simulink model "MPC_VSC_AS"  (R2022b)
settings: Solver=ode4  StartTime=0.0  StopTime=20  FixedStep=1e-3  RelTol=1e-3  EnableMultiTasking=on
values from neighbouring files (symbols this model uses):
  Dt = 0.01    [MAIN_AS.m]
  g = 9.81    [MAIN_AS.m]
  i_steer = 15.4    [MAIN_AS.m]
  Kus = m_f/Caf-m_r/Car    (= 0.00219239766082)    [MAIN_AS.m]
  L = 2.79    [MAIN_AS.m]
  mu = 1    [MAIN_AS.m]
  N = 20    [MAIN_AS.m]
  noise = 0    [MAIN_AS.m]
  tau = 0.09    [MAIN_AS.m]
  V_ref = 60/3.6    (= 16.6666666667)    [MAIN_AS.m]
  wn = 11    [MAIN_AS.m]
  xi = 0.7    [MAIN_AS.m]
undefined symbols (not defined in the file or in its folder): MPC_constraints, MPC_weights, par
libraries: simulink x2
settings Model: Creator=bshyrokau  LastModifiedBy=xippa
settings SolverCC: AlgebraicLoopSolver=TrustRegion
settings DataIOCC: SaveOutput=off  SignalLogging=off  DSMLogging=off  SaveTime=off  ReturnWorkspaceOutputs=off
settings OptimizationCC: LifeSpan=inf
settings DebuggingCC: UnconnectedInputMsg=warning  UnconnectedOutputMsg=warning  UnconnectedLineMsg=warning  AllowSymbolicDim=off  SFUnexpectedBacktrackingDiag=warning  SFNoUnconditionalDefaultTransitionDiag=warning  SFExecutionAtInitializationDiag=none  ArithmeticOperatorsInVariantConditions=warning
settings ModelReferenceCC: EnableRefExpFcnMdlSchedulingChecks=on  PropagateSignalLabelsOutOfModel=off
settings SFSimCC: SimUseLocalCustomCode=off  CustomCodeUndefinedFunction=UseInterfaceOnly
settings RTWCC: RTWUseLocalCustomCode=off  DLArmComputeVersion=19.05
settings CodeAppCC: StateflowObjectComments=on
settings GRTTargetCC: TargetLangStandard=C89/C90 (ANSI)
settings ConfigComp: CovMetricSettings=dw  CovSaveCumulativeToWorkspaceVar=on  CovSaveSingleToWorkspaceVar=on  CovExternalEMLEnable=off
settings SimscapeCC: SimscapeNormalizeSystem=off
settings ConfigurationSet: Description=SimMechanics 2G

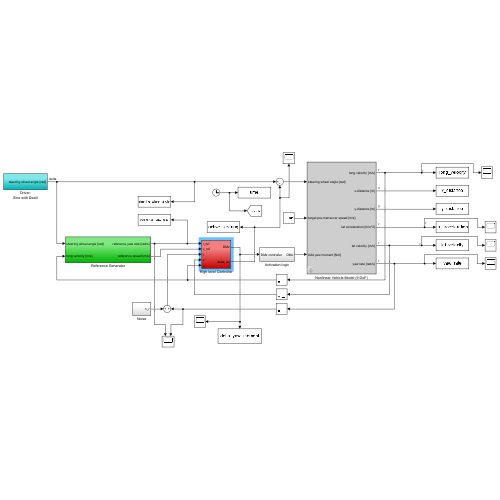
[thumbnail: Simulink's stored preview of the top-level diagram]
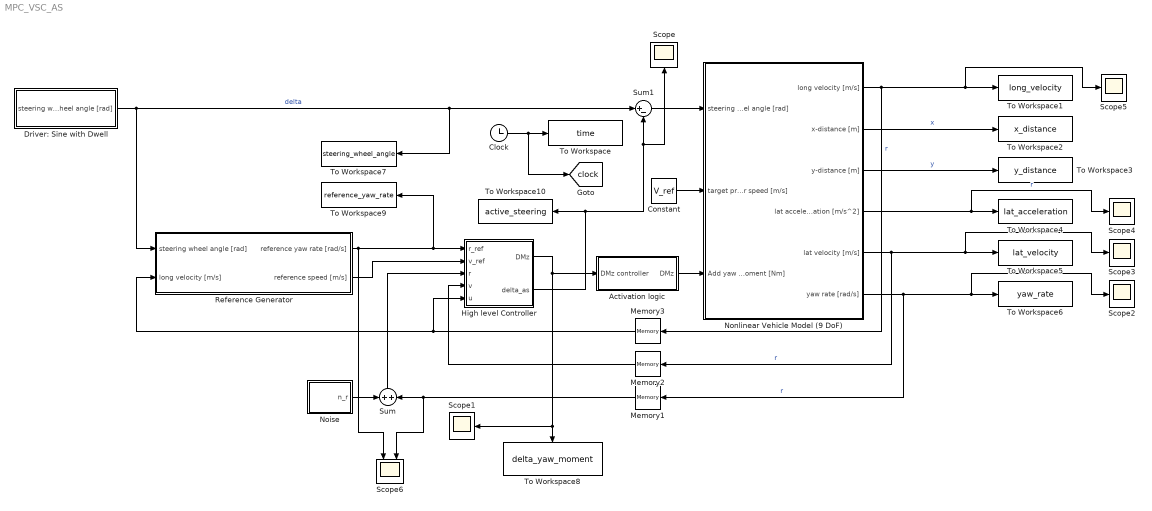
== system MPC_VSC_AS ==
  Activation logic : Subsystem
  Clock : Clock
  Constant : Constant  Value=V_ref
  Driver: Sine with Dwell : Subsystem
  High level Controller : Subsystem
  Memory1 : Memory
  Memory2 : Memory
  Memory3 : Memory
  Noise : Subsystem
  Nonlinear Vehicle Model (9 DoF) : Subsystem
      mask help: Simulink:masks:GenSFuncDesc_MD
      mask Help: eval('feval(''rtwprivate'',''rtwhelpview'',''rtw_sfcn_block'')');
  Reference Generator : Subsystem
  Scope{,1..5} (6 alike) : Scope
  Scope6 : Scope  NumInputPorts=2
  Sum : Sum  Inputs=+|+
  Sum1 : Sum  Inputs=|+-
  To Workspace : ToWorkspace  VariableName=time  SampleTime=-1
  To Workspace1 : ToWorkspace  VariableName=long_velocity  SampleTime=-1
  To Workspace10 : ToWorkspace  VariableName=active_steering  SampleTime=-1
  To Workspace2 : ToWorkspace  VariableName=x_distance  SampleTime=-1
  To Workspace3 : ToWorkspace  VariableName=y_distance  SampleTime=-1
  To Workspace4 : ToWorkspace  VariableName=lat_acceleration  SampleTime=-1
  To Workspace5 : ToWorkspace  VariableName=lat_velocity  SampleTime=-1
  To Workspace6 : ToWorkspace  VariableName=yaw_rate  SampleTime=-1
  To Workspace7 : ToWorkspace  VariableName=steering_wheel_angle  SampleTime=-1
  To Workspace8 : ToWorkspace  VariableName=delta_yaw_moment  SampleTime=-1
  To Workspace9 : ToWorkspace  VariableName=reference_yaw_rate  SampleTime=-1
  tag scope: clock=global
  wires:
  Driver: Sine with Dwell/1(steering wheel angle [rad]) -> Sum1/1, To Workspace7/1, Reference Generator/1(steering wheel angle [rad])  "delta"
  Reference Generator/1(reference yaw rate [rad/s]) -> High level Controller/1(r_ref), To Workspace9/1, Scope6/1
  Nonlinear Vehicle Model (9 DoF)/6(yaw rate [rad/s]) -> Scope2/1, To Workspace6/1, Memory1/1  "r"
  Nonlinear Vehicle Model (9 DoF)/2(x-distance [m]) -> To Workspace2/1  "x"
  Nonlinear Vehicle Model (9 DoF)/3(y-distance [m]) -> To Workspace3/1  "y"
  Constant/1 -> Nonlinear Vehicle Model (9 DoF)/2(target pre-maneuver speed [m/s])
  Clock/1 -> To Workspace/1, [clock]
  Memory1/1 -> Scope6/2, Sum/2
  Sum/1 -> High level Controller/3(r)
  Activation logic/1(DMz) -> Nonlinear Vehicle Model (9 DoF)/3(Add yaw moment [Nm])
  Noise/1(n_r) -> Sum/1
  Memory2/1 -> High level Controller/4(v)
  Memory3/1 -> High level Controller/5(u), Reference Generator/2(long velocity [m/s])
  Reference Generator/2(reference speed [m/s]) -> High level Controller/2(v_ref)
  High level Controller/1(DMz) -> Activation logic/1(DMz controller), Scope1/1, To Workspace8/1
  High level Controller/2(delta_as) -> To Workspace10/1, Scope/1, Sum1/2
  Sum1/1 -> Nonlinear Vehicle Model (9 DoF)/1(steering wheel angle [rad])
  Nonlinear Vehicle Model (9 DoF)/5(lat velocity [m/s]) -> Scope3/1, To Workspace5/1, Memory2/1  "r"
  Nonlinear Vehicle Model (9 DoF)/4(lat acceleration [m/s^2]) -> Scope4/1, To Workspace4/1  "r"
  Nonlinear Vehicle Model (9 DoF)/1(long velocity [m/s]) -> Scope5/1, To Workspace1/1, Memory3/1  "r"

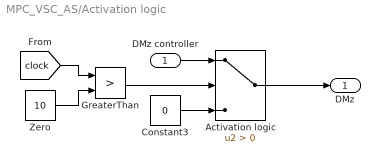
== system MPC_VSC_AS/Activation logic ==
  DMz controller : Inport
  Activation logic : Switch  Criteria=u2 > Threshold  SaturateOnIntegerOverflow=off  InputSameDT=off
  Constant3 : Constant  Value=0
  GreaterThan : RelationalOperator  Operator=>  OutDataTypeStr=boolean  RndMeth=Simplest  InputSameDT=off
  Zero : Constant  Value=10  OutDataTypeStr=Inherit: Inherit via back propagation
  DMz : Outport
  wires:
  [clock] -> GreaterThan/1
  GreaterThan/1 -> Activation logic/2
  Activation logic/1 -> DMz/1
  DMz controller/1 -> Activation logic/1
  Zero/1 -> GreaterThan/2
  Constant3/1 -> Activation logic/3

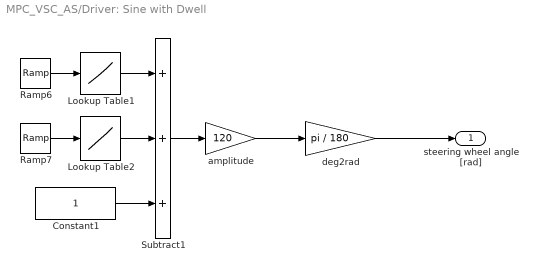
== system MPC_VSC_AS/Driver: Sine with Dwell ==
  Constant1 : Constant
  Lookup Table1 : Lookup  InputValues=[0:0.1:3*pi/2 3*pi/2+eps]*0.7  Table=sin([0:0.1:3*pi/2 3*pi/2+eps])  LookUpMeth=Interpolation-Use End Values  SaturateOnIntegerOverflow=off
  Lookup Table2 : Lookup  InputValues=[3*pi/2:0.1:2*pi 2*pi+eps]*0.7  Table=sin([3*pi/2:0.1:2*pi 2*pi+eps])  LookUpMeth=Interpolation-Use End Values  SaturateOnIntegerOverflow=off
  Ramp6 : simulink/Sources/Ramp  slope=pi  start=10  InitialOutput=0
  Ramp7 : simulink/Sources/Ramp  slope=pi  start=10+0.5  InitialOutput=0
  Subtract1 : Sum  Inputs=+++
  amplitude : Gain  Gain=120
  deg2rad : Gain  Gain=pi / 180
  steering wheel angle [rad] : Outport  VectorParamsAs1DForOutWhenUnconnected=off
  wires:
  Ramp6/1 -> Lookup Table1/1
  Ramp7/1 -> Lookup Table2/1
  Lookup Table2/1 -> Subtract1/2
  Lookup Table1/1 -> Subtract1/1
  Constant1/1 -> Subtract1/3
  Subtract1/1 -> amplitude/1
  amplitude/1 -> deg2rad/1
  deg2rad/1 -> steering wheel angle [rad]/1

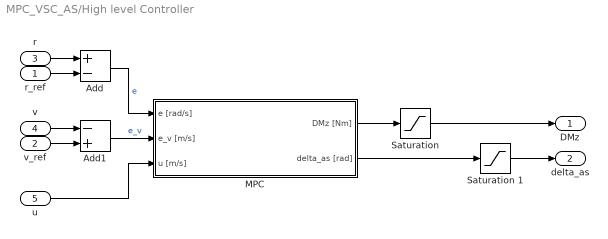
== system MPC_VSC_AS/High level Controller ==
  r_ref : Inport
  v_ref : Inport  Port=2
  r : Inport  Port=3
  v : Inport  Port=4
  u : Inport  Port=5
  Add : Sum  Inputs=+-
  Add1 : Sum  Inputs=-+
  MPC : Subsystem
  "Saturation " : Saturate  UpperLimit=10000  LowerLimit=-10000
  Saturation 1 : Saturate  UpperLimit=deg2rad(10)  LowerLimit=-deg2rad(10)
  DMz : Outport  VectorParamsAs1DForOutWhenUnconnected=off
  delta_as : Outport  Port=2  VectorParamsAs1DForOutWhenUnconnected=off
  wires:
  r_ref/1 -> Add/2
  "Saturation "/1 -> DMz/1
  Add/1 -> MPC/1(e [rad/s])  "e"
  r/1 -> Add/1
  v/1 -> Add1/1
  u/1 -> MPC/3(u [m/s])
  MPC/1(DMz [Nm]) -> "Saturation "/1
  v_ref/1 -> Add1/2
  Add1/1 -> MPC/2(e_v [m/s])  "e_v"
  MPC/2(delta_as [rad]) -> Saturation 1/1
  Saturation 1/1 -> delta_as/1

== system MPC_VSC_AS/Noise ==
  Constant1 : Constant  Value=0
  Constant2 : Constant  Value=noise
  Switch : Switch  Criteria=u2 > Threshold  SaturateOnIntegerOverflow=off  InputSameDT=off
  Uniform Random Number : UniformRandomNumber  Minimum=-deg2rad(0.5)  Maximum=deg2rad(0.5)  SampleTime=0.001
  n_r : Outport
  wires:
  Switch/1 -> n_r/1
  Constant2/1 -> Switch/2
  Constant1/1 -> Switch/3
  Uniform Random Number/1 -> Switch/1

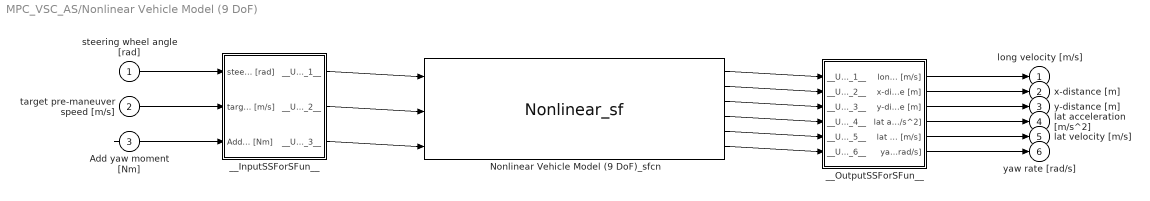
== system MPC_VSC_AS/Nonlinear Vehicle Model (9 DoF) ==
  steering wheel angle [rad] : Inport
  target pre-maneuver speed [m/s] : Inport  Port=2
  Add yaw moment [Nm] : Inport  Port=3
  Nonlinear Vehicle Model (9 DoF)_sfcn : S-Function  FunctionName=Nonlinear_sf  SFunctionModules=""  SFunctionDeploymentMode=off  EnableBusSupport=off  mask{rtw_sf_name=Nonlinear_sf, showVar=off}
      mask prompts: rtw_sf_name "Simulink:masks:GenSFuncName_MP"; showVar "Simulink:masks:GenSFuncShowModuleList_MP"
      mask help: Simulink:masks:GenSFuncDesc_MD
      mask init:
      | displist = '';
      | if ~strcmp(get_param(gcb, 'FunctionName'), rtw_sf_name);
      |   set_param(gcb, 'FunctionName', rtw_sf_name);
      | end
      | % Check if we are generating code
      | rtw_mode = false;
      | if strcmpi(get_param(bdroot(gcb),'SimulationStatus'),'Initializing')
      | 	rtw_mode = strcmpi(get_param(bdroot(gcb),'BuildingRTWCode'),'on') && ...
      | 		~strcmpi(get_param(bdroot(gcb),'TargetStyle'),'SimulationTarget');
      | end
      | if showVar || rtw_mode
      | 	if exist('rtwsfunc') == 2 | exist('rtwsfunc') == 6
      | 		tmplist = rtwsfunc(rtw_sf_name,gcb);
      | 		tmplist = DAStudio.message('Simulink:masks:GenSFuncListOfModules_IC', tmplist);
      | 	elseif showVar
      | 		tmplist1 = DAStudio.message('Simulink:masks:GenSFuncListOfModules_IC', '');
      |         tmplist2 = DAStudio.message('Simulink:masks:GenSFuncNotLicensed_IC');
      |         tmplist = [tmplist1 tmplist2];
      |  	end
      | end
      | if showVar
      |   displist = tmplist;
      | end
      settings: CopyFcn=|
      | if ~strcmp(get_param(gcb,'Linkstatus'),'none') && ...
      | ~strcmp(get_param(gcb,'Linkstatus'),'implicit')
      |   set_param(gcb,'LinkStatus','none');
      | end
      mask Help: eval('feval(''rtwprivate'',''rtwhelpview'',''rtw_sfcn_block'')');
      mask Display:
      | port_label('input',1,'steering wheel angle [rad]');
      | port_label('input',2,'target pre-maneuver speed [m/s]');
      | port_label('input',3,'Add yaw moment [Nm]');
      | port_label('output',1,'long velocity [m/s]');
      | port_label('output',2,'x-distance [m]');
      | port_label('output',3,'y-distance [m]');
      | port_label('output',4,'lat acceleration [m/s^2]');
      | port_label('output',5,'lat velocity [m/s]');
      | port_label('output',6,'yaw rate [rad/s]');
  __InputSSForSFun__ : Subsystem
  __OutputSSForSFun__ : Subsystem
  long velocity [m/s] : Outport  VectorParamsAs1DForOutWhenUnconnected=off
  x-distance [m] : Outport  Port=2  VectorParamsAs1DForOutWhenUnconnected=off
  y-distance [m] : Outport  Port=3  VectorParamsAs1DForOutWhenUnconnected=off
  lat acceleration [m/s^2] : Outport  Port=4  VectorParamsAs1DForOutWhenUnconnected=off
  lat velocity [m/s] : Outport  Port=5  VectorParamsAs1DForOutWhenUnconnected=off
  yaw rate [rad/s] : Outport  Port=6  VectorParamsAs1DForOutWhenUnconnected=off
  wires:
  steering wheel angle [rad]/1 -> __InputSSForSFun__/1(steering wheel angle [rad])
  target pre-maneuver speed [m/s]/1 -> __InputSSForSFun__/2(target pre-maneuver speed [m/s])
  Add yaw moment [Nm]/1 -> __InputSSForSFun__/3(Add yaw moment [Nm])
  __InputSSForSFun__/1(__UniqueOutportName__1__) -> Nonlinear Vehicle Model (9 DoF)_sfcn/1
  __InputSSForSFun__/2(__UniqueOutportName__2__) -> Nonlinear Vehicle Model (9 DoF)_sfcn/2
  __InputSSForSFun__/3(__UniqueOutportName__3__) -> Nonlinear Vehicle Model (9 DoF)_sfcn/3
  Nonlinear Vehicle Model (9 DoF)_sfcn/1 -> __OutputSSForSFun__/1(__UniqueInportName__1__)
  Nonlinear Vehicle Model (9 DoF)_sfcn/2 -> __OutputSSForSFun__/2(__UniqueInportName__2__)
  Nonlinear Vehicle Model (9 DoF)_sfcn/3 -> __OutputSSForSFun__/3(__UniqueInportName__3__)
  Nonlinear Vehicle Model (9 DoF)_sfcn/4 -> __OutputSSForSFun__/4(__UniqueInportName__4__)
  Nonlinear Vehicle Model (9 DoF)_sfcn/5 -> __OutputSSForSFun__/5(__UniqueInportName__5__)
  Nonlinear Vehicle Model (9 DoF)_sfcn/6 -> __OutputSSForSFun__/6(__UniqueInportName__6__)
  __OutputSSForSFun__/1(long velocity [m/s]) -> long velocity [m/s]/1
  __OutputSSForSFun__/2(x-distance [m]) -> x-distance [m]/1
  __OutputSSForSFun__/3(y-distance [m]) -> y-distance [m]/1
  __OutputSSForSFun__/4(lat acceleration [m/s^2]) -> lat acceleration [m/s^2]/1
  __OutputSSForSFun__/5(lat velocity [m/s]) -> lat velocity [m/s]/1
  __OutputSSForSFun__/6(yaw rate [rad/s]) -> yaw rate [rad/s]/1

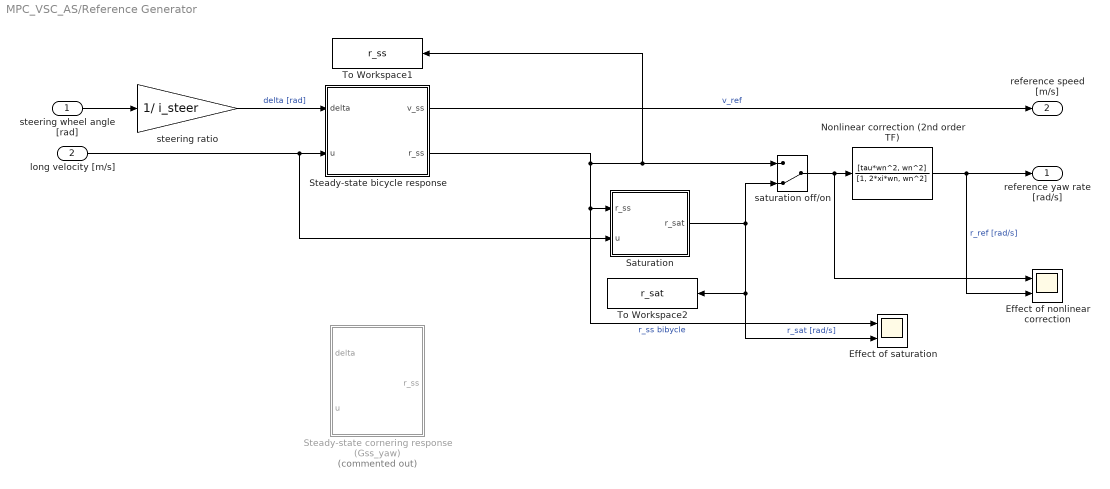
== system MPC_VSC_AS/Reference Generator ==
  steering wheel angle [rad] : Inport
  long velocity [m/s] : Inport  Port=2
  Effect of nonlinear correction : Scope  NumInputPorts=2
  Effect of saturation : Scope  NumInputPorts=2
  Nonlinear correction (2nd order TF) : TransferFcn  Numerator=[tau*wn^2, wn^2]  Denominator=[1, 2*xi*wn, wn^2]
  Saturation : Subsystem
  Steady-state bicycle response : MATLAB Function  TreatAsAtomicUnit=on
  Steady-state cornering response (Gss_yaw) : Subsystem  Commented=on
  To Workspace1 : ToWorkspace  VariableName=r_ss  SampleTime=-1
  To Workspace2 : ToWorkspace  VariableName=r_sat  SampleTime=-1
  saturation off/on : ManualSwitch  CurrentSetting=0
  steering ratio : Gain  Gain=1/ i_steer
  reference yaw rate [rad/s] : Outport  VectorParamsAs1DForOutWhenUnconnected=off
  reference speed [m/s] : Outport  Port=2  VectorParamsAs1DForOutWhenUnconnected=off
  wires:
  steering wheel angle [rad]/1 -> steering ratio/1
  steering ratio/1 -> Steady-state bicycle response/1(delta)  "delta [rad]"
  Steady-state bicycle response/2(r_ss) -> To Workspace1/1, saturation off/on/1, Effect of saturation/1, Saturation/1(r_ss)  "r_ss bibycle"
  Nonlinear correction (2nd order TF)/1 -> Effect of nonlinear correction/2, reference yaw rate [rad/s]/1  "r_ref [rad/s]"
  Saturation/1(r_sat) -> Effect of saturation/2, To Workspace2/1, saturation off/on/2  "r_sat [rad/s]"
  long velocity [m/s]/1 -> Saturation/2(u), Steady-state bicycle response/2(u)
  Steady-state bicycle response/1(v_ss) -> reference speed [m/s]/1  "v_ref"
  saturation off/on/1 -> Effect of nonlinear correction/1, Nonlinear correction (2nd order TF)/1

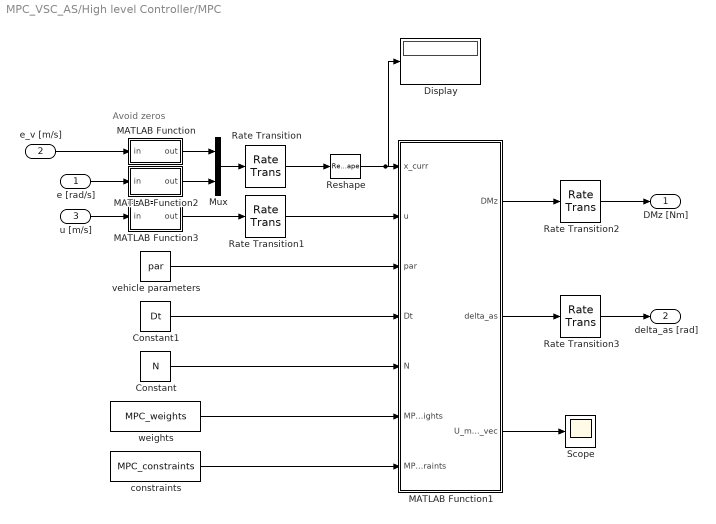
== system MPC_VSC_AS/High level Controller/MPC ==
  note: Avoid zeros
  e [rad/s] : Inport
  e_v [m/s] : Inport  Port=2
  u [m/s] : Inport  Port=3
  Constant : Constant  Value=N
  Constant1 : Constant  Value=Dt
  Display : Display
  MATLAB Function : MATLAB Function  TreatAsAtomicUnit=on
  MATLAB Function1 : MATLAB Function  TreatAsAtomicUnit=on
  MATLAB Function2 : MATLAB Function  TreatAsAtomicUnit=on
  MATLAB Function3 : MATLAB Function  TreatAsAtomicUnit=on
  Mux : Mux  Inputs=2
  Rate Transition : RateTransition  OutPortSampleTime=Dt
  Rate Transition1 : RateTransition  OutPortSampleTime=Dt
  Rate Transition2 : RateTransition  OutPortSampleTime=1e-3
  Rate Transition3 : RateTransition  OutPortSampleTime=1e-3
  Reshape : Reshape  OutputDimensionality=Customize  OutputDimensions=[2,1]
  Scope : Scope
  constraints : Constant  Value=MPC_constraints  OutDataTypeStr=Bus: constraintsBus
  vehicle parameters : Constant  Value=par  OutDataTypeStr=Bus: parBus
  weights : Constant  Value=MPC_weights  OutDataTypeStr=Bus: weightsBus
  DMz [Nm] : Outport
  delta_as [rad] : Outport  Port=2
  wires:
  e [rad/s]/1 -> MATLAB Function2/1(in)
  MATLAB Function1/1(DMz) -> Rate Transition2/1
  e_v [m/s]/1 -> MATLAB Function/1(in)
  Mux/1 -> Rate Transition/1
  vehicle parameters/1 -> MATLAB Function1/3(par)
  Constant/1 -> MATLAB Function1/5(N)
  Constant1/1 -> MATLAB Function1/4(Dt)
  u [m/s]/1 -> MATLAB Function3/1(in)
  weights/1 -> MATLAB Function1/6(MPC_weights)
  constraints/1 -> MATLAB Function1/7(MPC_constraints)
  Rate Transition1/1 -> MATLAB Function1/2(u)
  Rate Transition2/1 -> DMz [Nm]/1
  MATLAB Function/1(out) -> Mux/1
  MATLAB Function2/1(out) -> Mux/2
  MATLAB Function3/1(out) -> Rate Transition1/1
  Rate Transition3/1 -> delta_as [rad]/1
  MATLAB Function1/2(delta_as) -> Rate Transition3/1
  Rate Transition/1 -> Reshape/1
  Reshape/1 -> Display/1, MATLAB Function1/1(x_curr)
  MATLAB Function1/3(U_min_vec) -> Scope/1

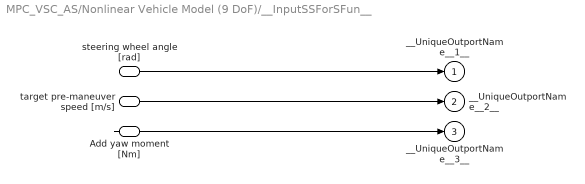
== system MPC_VSC_AS/Nonlinear Vehicle Model (9 DoF)/__InputSSForSFun__ ==
  steering wheel angle [rad] : Inport
  target pre-maneuver speed [m/s] : Inport  Port=2
  Add yaw moment [Nm] : Inport  Port=3
  __UniqueOutportName__1__ : Outport
  __UniqueOutportName__2__ : Outport  Port=2
  __UniqueOutportName__3__ : Outport  Port=3
  wires:
  steering wheel angle [rad]/1 -> __UniqueOutportName__1__/1
  target pre-maneuver speed [m/s]/1 -> __UniqueOutportName__2__/1
  Add yaw moment [Nm]/1 -> __UniqueOutportName__3__/1

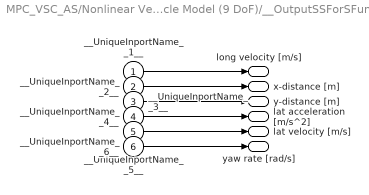
== system MPC_VSC_AS/Nonlinear Vehicle Model (9 DoF)/__OutputSSForSFun__ ==
  __UniqueInportName__1__ : Inport
  __UniqueInportName__2__ : Inport  Port=2
  __UniqueInportName__3__ : Inport  Port=3
  __UniqueInportName__4__ : Inport  Port=4
  __UniqueInportName__5__ : Inport  Port=5
  __UniqueInportName__6__ : Inport  Port=6
  long velocity [m/s] : Outport  VectorParamsAs1DForOutWhenUnconnected=off
  x-distance [m] : Outport  Port=2  VectorParamsAs1DForOutWhenUnconnected=off
  y-distance [m] : Outport  Port=3  VectorParamsAs1DForOutWhenUnconnected=off
  lat acceleration [m/s^2] : Outport  Port=4  VectorParamsAs1DForOutWhenUnconnected=off
  lat velocity [m/s] : Outport  Port=5  VectorParamsAs1DForOutWhenUnconnected=off
  yaw rate [rad/s] : Outport  Port=6  VectorParamsAs1DForOutWhenUnconnected=off
  wires:
  __UniqueInportName__1__/1 -> long velocity [m/s]/1
  __UniqueInportName__2__/1 -> x-distance [m]/1
  __UniqueInportName__3__/1 -> y-distance [m]/1
  __UniqueInportName__4__/1 -> lat acceleration [m/s^2]/1
  __UniqueInportName__5__/1 -> lat velocity [m/s]/1
  __UniqueInportName__6__/1 -> yaw rate [rad/s]/1

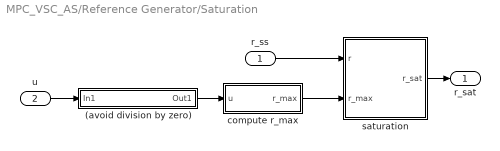
== system MPC_VSC_AS/Reference Generator/Saturation ==
  r_ss : Inport
  u : Inport  Port=2
  (avoid division by zero) : Subsystem
  compute r_max : Subsystem
  saturation : MATLAB Function  TreatAsAtomicUnit=on
  r_sat : Outport
  wires:
  compute r_max/1(r_max) -> saturation/2(r_max)
  saturation/1(r_sat) -> r_sat/1
  r_ss/1 -> saturation/1(r)
  u/1 -> (avoid division by zero)/1(In1)
  (avoid division by zero)/1(Out1) -> compute r_max/1(u)

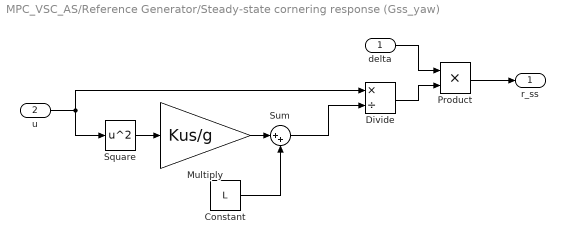
== system MPC_VSC_AS/Reference Generator/Steady-state cornering response (Gss_yaw) ==
  delta : Inport
  u : Inport  Port=2
  Constant : Constant  Value=L
  Divide : Product  Inputs=*/
  Multiply : Gain  Gain=Kus/g
  Product : Product
  Square : Math  Operator=square
  Sum : Sum  Inputs=|++
  r_ss : Outport
  wires:
  u/1 -> Square/1, Divide/1
  Square/1 -> Multiply/1
  Multiply/1 -> Sum/1
  Constant/1 -> Sum/2
  Sum/1 -> Divide/2
  delta/1 -> Product/1
  Divide/1 -> Product/2
  Product/1 -> r_ss/1

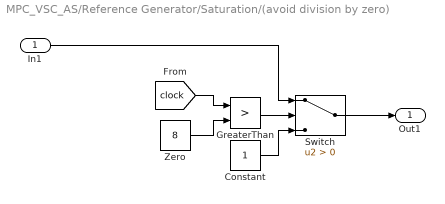
== system MPC_VSC_AS/Reference Generator/Saturation/(avoid division by zero) ==
  In1 : Inport
  Constant : Constant
  GreaterThan : RelationalOperator  Operator=>  OutDataTypeStr=boolean  RndMeth=Simplest  InputSameDT=off
  Switch : Switch  Criteria=u2 > Threshold  SaturateOnIntegerOverflow=off  InputSameDT=off
  Zero : Constant  Value=8  OutDataTypeStr=Inherit: Inherit via back propagation
  Out1 : Outport
  wires:
  Constant/1 -> Switch/3
  [clock] -> GreaterThan/1
  GreaterThan/1 -> Switch/2
  Switch/1 -> Out1/1
  In1/1 -> Switch/1
  Zero/1 -> GreaterThan/2

== system MPC_VSC_AS/Reference Generator/Saturation/compute r_max ==
  u : Inport
  Constant : Constant  Value=0.85*mu*g
  Divide : Product  Inputs=*/
  r_max : Outport
  wires:
  Constant/1 -> Divide/1
  Divide/1 -> r_max/1
  u/1 -> Divide/2

== matlab function MPC_VSC_AS/Reference Generator/Steady-state bicycle response ==
  data: v_ss output; delta input; u input; r_ss output
function [v_ss,r_ss]=ssBicycle(delta,u)

% Parameters
m = 1380;       % vehicle mass [Kg]    
L = 2.79;       % wheelbase [m]
lf = 1.384;     % distance from front axle to CoG [m]
lr = L-lf;      % distance from rear axle to CoG [m]
Caf = 120000;   % front axle cornering stiffness
Car = 190000;   % rear axle cornering stiffness
Iz = 2634.5;    % body inertia around z-axis [Kg m^2]

% Compute A matrix
A=zeros(2,2);
A(1,1)=-(Caf+Car)/(m*u);
A(1,2)=(lr*Car-lf*Caf)/(m*u)-u;
A(2,1)=(lr*Car-lf*Caf)/(Iz*u);
A(2,2)=-(lf^2*Caf+lr^2*Car)/(Iz*u);

% Compute B vector
B=[Caf/m Caf*lf/Iz]';

% Solve steady-state bicycle
x_ref=-A\(B*delta);
v_ss=x_ref(1);
r_ss=x_ref(2);

if any(isnan(x_ref))
    v_ss=0;
    r_ss=0;
end

end

== matlab function MPC_VSC_AS/Reference Generator/Saturation/saturation ==
  data: r input; r_sat output; r_max input
function r_sat=sat(r,r_max)

if r>r_max
    r_sat=r_max;
elseif r<-r_max
    r_sat=-r_max;
else
    r_sat=r;
end

end

== matlab function MPC_VSC_AS/High level Controller/MPC/MATLAB Function ==
  data: in input; out output
function out=fcn(in)

if in==0
    out=0.001;
else
    out=in;
end

end

== matlab function MPC_VSC_AS/High level Controller/MPC/MATLAB Function1 ==
  data: x_curr input; u input; par input; Dt input; DMz output; N input; MPC_weights input; MPC_constraints input; delta_as output; U_min_vec output
function [DMz, delta_as, U_min_vec] = MPC(x_curr,u,par,Dt,N,MPC_weights,MPC_constraints)
% Extract relevant parameters from structs
Iz=par.Iz;
Caf=par.Caf;
lf=par.lf;
m=par.m;
Q=MPC_weights.Q;
R=MPC_weights.R;
P=MPC_weights.P;
U_min=MPC_constraints.U_min;
U_max=MPC_constraints.U_max;
x_min=MPC_constraints.x_min;
x_max=MPC_constraints.x_max;

% Compute Ad and BMd matrices
A=ComputeA(u,par);
BM=[0, Caf*lf/m;
 1/Iz, Caf*lf/Iz];
[Ad,Bd]=ComputeDiscretizedMatrices(A,BM,Dt);

% Compute prediction matrices
[T,S]=PredMatGen(Ad,Bd,eye(2),N);

% Compute cost function matrices
[H,h]=CostFuncGen(T,S,Q,R,P);

% Compute state constraints
A_tilde=[Ad; -Ad];
B_tilde=[Bd; -Bd];
A_bar=kron(eye(N),A_tilde);
B_bar=kron(eye(N),B_tilde);
A_ineq=A_bar*S(1:end-2,:)+B_bar;
b_tilde=[x_max; -x_min];
b_bar=repmat(b_tilde,N,1);
b_ineq=b_bar-A_bar*T(1:end-2,:)*x_curr;

U_min_vec = reshape(U_min', [], 1);
U_max_vec = reshape(U_max', [], 1);
U0 = (U_min_vec + U_max_vec) / 2;

% quadprog solver for optimization
options=optimoptions('quadprog','Algorithm','active-set');
[U_opt,~,~] = quadprog(H, h * x_curr, A_ineq, b_ineq, [], [], U_min_vec, U_max_vec, U0, options);
DMz = U_opt(1);
delta_as = U_opt(2);
DMz = double(DMz);
delta_as = double(delta_as);

end

== matlab function MPC_VSC_AS/High level Controller/MPC/MATLAB Function2 ==
  data: in input; out output
function out=fcn(in)

if in==0
    out=0.001;
else
    out=in;
end

end

== matlab function MPC_VSC_AS/High level Controller/MPC/MATLAB Function3 ==
  data: in input; out output
function out=fcn(in)

if in==0
    out=0.001;
else
    out=in;
end

end
